simulink model "lab2_0x2810x29"  (R2024a)
settings: Solver=ode23t  StartTime=0.0  StopTime=1  RelTol=1e-3
libraries: dspfdesign x6
settings Model: Creator=CS Net Games  LastModifiedBy=hp
settings SolverCC: AlgebraicLoopSolver=TrustRegion
settings DebuggingCC: UnconnectedInputMsg=warning  UnconnectedOutputMsg=warning  UnconnectedLineMsg=warning
settings ModelReferenceCC: EnableRefExpFcnMdlSchedulingChecks=on
settings SFSimCC: CustomCodeUndefinedFunction=UseInterfaceOnly
settings RTWCC: GPUComputeCapability=3.5

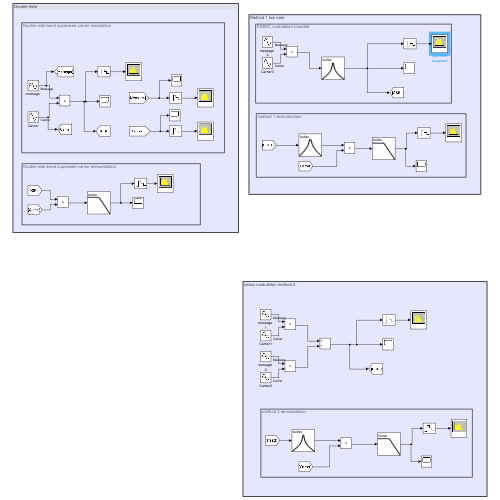
[thumbnail: Simulink's stored preview of the top-level diagram]
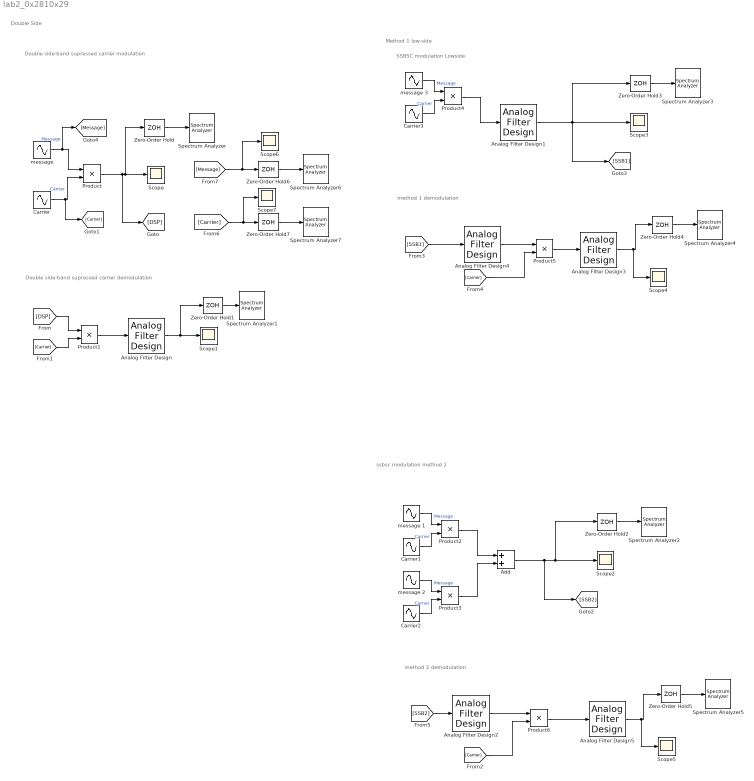
== system lab2_0x2810x29 ==
  note: Double side-band supressed carrier demodulation
  note: Double side-band supressed carrier modulation
  note: method 1 demodulation
  note: SSBSC modulation Lowside
  note: method 2 demodulation
  note: ssbsc modulation method 2
  note: Method 1 low-side
  note: Double Side
  Add : Sum
  Analog Filter Design : dspfdesign/Analog Filter Design  method=Butterworth  filttype=Lowpass  N=8  Wlo=pi*2*1200  Whi=80  Rp=2  Rs=40
  Analog Filter Design1 : dspfdesign/Analog Filter Design  method=Butterworth  filttype=Bandpass  N=8  Wlo=pi*2*13000  Whi=pi*2*15000  Rp=2  Rs=40
  Analog Filter Design2 : dspfdesign/Analog Filter Design  method=Butterworth  filttype=Bandpass  N=8  Wlo=pi*2*13000  Whi=pi*2*15000  Rp=2  Rs=40
  Analog Filter Design3 : dspfdesign/Analog Filter Design  method=Butterworth  filttype=Lowpass  N=8  Wlo=pi*2*1200  Whi=80  Rp=2  Rs=40
  Analog Filter Design4 : dspfdesign/Analog Filter Design  method=Butterworth  filttype=Bandpass  N=8  Wlo=pi*2*13000  Whi=pi*2*17000  Rp=2  Rs=40
  Analog Filter Design5 : dspfdesign/Analog Filter Design  method=Butterworth  filttype=Lowpass  N=8  Wlo=pi*2*1500  Whi=80  Rp=2  Rs=40
  Carrier{,1..3} (4 alike) : Sin  Frequency=pi*2*15000  SampleTime=0
  Product{,1..6} (7 alike) : Product
  Scope{,1..7} (8 alike) : Scope
  Spectrum Analyzer : SpectrumAnalyzer  WindowPosition=[1.000000,1.000000,1280.000000,697.000000,]  ScopeFrameLocation=window  SpectrumType=RMS  Method=Welch  SampleRate=150000  AxesScaling=Manual  Span=150000  StartFrequency=-75000  StopFrequency=75000  AveragingMethod=Running  SpectrumUnits=Vrms  YLimits=[-0.026127601930479721348,0.23514841919442297513]  ShowLegend=on  ChannelNames="[\"modulated signal\"]"  AllowFFTLengthLessThanSamplesPerUpdate=on  DefaultConfigurationName=spbscopes.SpectrumAnalyzerBlockCfg  IsFrequencyInputMode=0  FrequencyVectorPort=0  FrequencyVectorFromPort=0  FrequencyInputRBWPort=0  FrequencyInputRBWFromPort=0
      settings: OpenAtSimulationStart=off
  Spectrum Analyzer1 : SpectrumAnalyzer  WindowPosition=[1.000000,1.000000,1280.000000,697.000000,]  ScopeFrameLocation=window  SpectrumType=RMS  Method=Welch  AxesScaling=Manual  AveragingMethod=Running  SpectrumUnits=Vrms  YLimits=[-0.023914219367317544884,0.21522797619659583823]  ShowLegend=on  ChannelNames="[\"demodulated signal\"]"  AllowFFTLengthLessThanSamplesPerUpdate=on  DefaultConfigurationName=spbscopes.SpectrumAnalyzerBlockCfg  IsFrequencyInputMode=0  FrequencyVectorPort=0  FrequencyVectorFromPort=0  FrequencyInputRBWPort=0  FrequencyInputRBWFromPort=0
      settings: OpenAtSimulationStart=off
  Spectrum Analyzer2 : SpectrumAnalyzer  WindowPosition=[1.000000,1.000000,1280.000000,697.000000,]  ScopeFrameLocation=window  SpectrumType=RMS  Method=Welch  SampleRate=150000  AxesScaling=Manual  Span=150000  StartFrequency=-75000  StopFrequency=75000  AveragingMethod=Running  SpectrumUnits=Vrms  YLimits=[-0.052253348060846652179,0.4702801389579952529]  ShowLegend=on  ChannelNames="[\"modulated single side\"]"  AllowFFTLengthLessThanSamplesPerUpdate=on  DefaultConfigurationName=spbscopes.SpectrumAnalyzerBlockCfg  IsFrequencyInputMode=0  FrequencyVectorPort=0  FrequencyVectorFromPort=0  FrequencyInputRBWPort=0  FrequencyInputRBWFromPort=0
      settings: OpenAtSimulationStart=off
  Spectrum Analyzer3 : SpectrumAnalyzer  WindowPosition=[-128.000000,-14.000000,1282.000000,700.000000,]  ScopeFrameLocation=window  SpectrumType=RMS  Method=Welch  SampleRate=150000  Span=150000  StartFrequency=-75000  StopFrequency=75000  AveragingMethod=Running  SpectrumUnits=Vrms  YLimits=[-0.02441151,0.21970362]  ShowLegend=on  ChannelNames="[\"Single side supressed carrier \"]"  AllowFFTLengthLessThanSamplesPerUpdate=on  DefaultConfigurationName=spbscopes.SpectrumAnalyzerBlockCfg  IsFrequencyInputMode=0  FrequencyVectorPort=0  FrequencyVectorFromPort=0  FrequencyInputRBWPort=0  FrequencyInputRBWFromPort=0
      settings: OpenAtSimulationStart=off
  Spectrum Analyzer4 : SpectrumAnalyzer  WindowPosition=[1.000000,1.000000,1280.000000,697.000000,]  ScopeFrameLocation=window  SpectrumType=RMS  Method=Welch  SampleRate=150000  AxesScaling=Manual  Span=150000  StartFrequency=-75000  StopFrequency=75000  AveragingMethod=Running  SpectrumUnits=Vrms  YLimits=[-0.012458084977529709433,0.11212276483722737053]  ShowLegend=on  ChannelNames="[\"demodulated signal\"]"  AllowFFTLengthLessThanSamplesPerUpdate=on  DefaultConfigurationName=spbscopes.SpectrumAnalyzerBlockCfg  IsFrequencyInputMode=0  FrequencyVectorPort=0  FrequencyVectorFromPort=0  FrequencyInputRBWPort=0  FrequencyInputRBWFromPort=0
      settings: OpenAtSimulationStart=off
  Spectrum Analyzer5 : SpectrumAnalyzer  WindowPosition=[1.000000,1.000000,1280.000000,697.000000,]  ScopeFrameLocation=window  SpectrumType=RMS  Method=Welch  SampleRate=150000  AxesScaling=Manual  Span=150000  StartFrequency=-75000  StopFrequency=75000  AveragingMethod=Running  SpectrumUnits=Vrms  YLimits=[-0.025479003903654467295,0.22931103517174417084]  ShowLegend=on  ChannelNames="[\"demodulated signal\"]"  AllowFFTLengthLessThanSamplesPerUpdate=on  DefaultConfigurationName=spbscopes.SpectrumAnalyzerBlockCfg  IsFrequencyInputMode=0  FrequencyVectorPort=0  FrequencyVectorFromPort=0  FrequencyInputRBWPort=0  FrequencyInputRBWFromPort=0
      settings: OpenAtSimulationStart=off
  Spectrum Analyzer6 : SpectrumAnalyzer  WindowPosition=[1.000000,1.000000,1280.000000,697.000000,]  ScopeFrameLocation=window  SpectrumType=RMS  Method=Welch  AxesScaling=Manual  AveragingMethod=Running  SpectrumUnits=Vrms  YLimits=[-0.047864785119498619304,0.43078306607548871865]  ShowLegend=on  ChannelNames="[\"message in frequency \"]"  AllowFFTLengthLessThanSamplesPerUpdate=on  DefaultConfigurationName=spbscopes.SpectrumAnalyzerBlockCfg  IsFrequencyInputMode=0  FrequencyVectorPort=0  FrequencyVectorFromPort=0  FrequencyInputRBWPort=0  FrequencyInputRBWFromPort=0
      settings: OpenAtSimulationStart=off
  Spectrum Analyzer7 : SpectrumAnalyzer  WindowPosition=[-128.000000,-14.000000,1282.000000,700.000000,]  ScopeFrameLocation=window  SpectrumType=RMS  Method=Welch  SampleRate=150000  AxesScaling=Manual  Span=150000  StartFrequency=-75000  StopFrequency=75000  AveragingMethod=Running  SpectrumUnits=Vrms  YLimits=[-0.056311512071850283734,0.5068036174957696316]  ShowLegend=on  ChannelNames="[\"Carrier in Frequency\"]"  AllowFFTLengthLessThanSamplesPerUpdate=on  DefaultConfigurationName=spbscopes.SpectrumAnalyzerBlockCfg  IsFrequencyInputMode=0  FrequencyVectorPort=0  FrequencyVectorFromPort=0  FrequencyInputRBWPort=0  FrequencyInputRBWFromPort=0
      settings: OpenAtSimulationStart=off
  Zero-Order Hold : ZeroOrderHold  SampleTime=1/(10*15e3)
  Zero-Order Hold1 : ZeroOrderHold  SampleTime=1/(10*1e3)
  Zero-Order Hold{2..5,7} (5 alike) : ZeroOrderHold  SampleTime=-1
  Zero-Order Hold6 : ZeroOrderHold  SampleTime=1/(10*1e3)
  message {,1..3} (4 alike) : Sin  Amplitude=0.85  Frequency=pi*2*1000  SampleTime=0
  wires:
  Product2/1 -> Add/1
  message 2/1 -> Product3/1  "Message"
  Carrier2/1 -> Product3/2  "Carrier"
  Product3/1 -> Add/2
  Carrier1/1 -> Product2/2  "Carrier"
  Zero-Order Hold2/1 -> Spectrum Analyzer2/1
  Add/1 -> Zero-Order Hold2/1, Scope2/1, [SSB2]
  message 1/1 -> Product2/1  "Message"
  Analog Filter Design5/1 -> Zero-Order Hold5/1, Scope5/1
  Analog Filter Design2/1 -> Product6/1
  [Carrier] -> Product6/2
  Product6/1 -> Analog Filter Design5/1
  Zero-Order Hold5/1 -> Spectrum Analyzer5/1
  [SSB2] -> Analog Filter Design2/1
  Carrier3/1 -> Product4/2  "Carrier"
  Product4/1 -> Analog Filter Design1/1
  message 3/1 -> Product4/1  "Message"
  Zero-Order Hold3/1 -> Spectrum Analyzer3/1
  Analog Filter Design1/1 -> Scope3/1, Zero-Order Hold3/1, [SSB1]
  Product5/1 -> Analog Filter Design3/1
  [SSB1] -> Analog Filter Design4/1
  [Carrier] -> Product5/2
  Zero-Order Hold4/1 -> Spectrum Analyzer4/1
  Analog Filter Design4/1 -> Product5/1
  Analog Filter Design3/1 -> Zero-Order Hold4/1, Scope4/1
  Zero-Order Hold/1 -> Spectrum Analyzer/1
  Zero-Order Hold7/1 -> Spectrum Analyzer7/1
  [Message] -> Scope6/1, Zero-Order Hold6/1
  Carrier/1 -> Product/2, [Carrier]  "Carrier"
  Zero-Order Hold6/1 -> Spectrum Analyzer6/1
  Product/1 -> Scope/1, Zero-Order Hold/1, [DSP]
  [Carrier] -> Scope7/1, Zero-Order Hold7/1
  "message "/1 -> [Message], Product/1  "Message"
  [DSP] -> Product1/1
  Product1/1 -> Analog Filter Design/1
  Zero-Order Hold1/1 -> Spectrum Analyzer1/1
  Analog Filter Design/1 -> Scope1/1, Zero-Order Hold1/1
  [Carrier] -> Product1/2
